simulink model "softpl1"  (Simulink 2.20)
settings: Solver=ode45  StartTime=0.0  StopTime=10  MaxStep=0.01  RelTol=1e-4  AbsTol=1e-4
settings Model: TimeSaveName=t  SaveOutput=off  ConsistencyChecking=off  RTWPlaceOutputsASAP=off

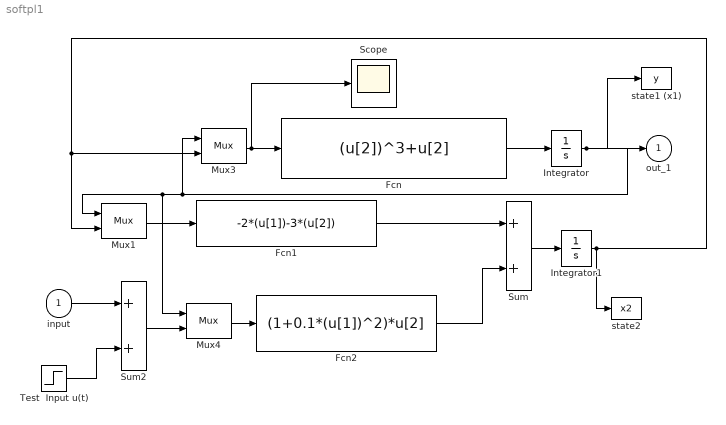
== system softpl1 ==
  input : Inport  Port=1  PortWidth=-1  SampleTime=-1
  Fcn : Fcn  Expr=(u[2])^3+u[2]
  Fcn1 : Fcn  Expr=-2*(u[1])-3*(u[2])
  Fcn2 : Fcn  Expr=(1+0.1*(u[1])^2)*u[2]
  Integrator : Integrator  ExternalReset=none  InitialConditionSource=internal  InitialCondition=0  LimitOutput=off  UpperSaturationLimit=inf  LowerSaturationLimit=-inf  ShowSaturationPort=off  ShowStatePort=off  AbsoluteTolerance=auto
  Integrator1 : Integrator  ExternalReset=none  InitialConditionSource=internal  InitialCondition=0  LimitOutput=off  UpperSaturationLimit=inf  LowerSaturationLimit=-inf  ShowSaturationPort=off  ShowStatePort=off  AbsoluteTolerance=auto
  Mux1 : Mux  Inputs=2
  Mux3 : Mux  Inputs=2
  Mux4 : Mux  Inputs=2
  Scope : Scope
      settings: TickLabels=on  TimeRange=20.000000  YMin=-2.000000  YMax=2.000000  SaveToWorkspace=off  SaveName=ScopeData
  Sum : Sum  Inputs=++
  Sum2 : Sum  Inputs=++
  Test  Input u(t) : Step  Time=1  Before=0  After=1
  state1 (x1) : ToWorkspace  VariableName=y  SampleTime=0
      settings: Buffer=20000
  state2 : ToWorkspace  VariableName=x2  SampleTime=0
      settings: Buffer=20000
  out_1 : Outport  Port=1  InitialOutput=0
  wires:
  Integrator1/1 -> state2/1, Mux1/2, Mux3/2
  Integrator/1 -> out_1/1, state1 (x1)/1, Mux1/1, Mux4/1, Mux3/1
  Mux4/1 -> Fcn2/1
  Fcn2/1 -> Sum/2
  Sum/1 -> Integrator1/1
  Fcn1/1 -> Sum/1
  Mux1/1 -> Fcn1/1
  Fcn/1 -> Integrator/1
  Sum2/1 -> Mux4/2
  input/1 -> Sum2/1
  Test  Input u(t)/1 -> Sum2/2
  Mux3/1 -> Fcn/1, Scope/1
